simulink model "Questao6_lab3_d"  (R2022b)
settings: Solver=VariableStepAuto  StartTime=0.0  StopTime=43200  RelTol=1e-3
model workspace (MAT data in the model file):
  Cc = 144870
  Ce = 132.0152
  Ci = 959.0196
  Rai = 10.1213
  Rca = 0.0037
  Rcp = 0.0021
  Rec = 0.7046
  Rei = 0.3194
  gamma = 0.021
libraries: simulink x1
settings Model: Creator=pedro  LastModifiedBy=pedro

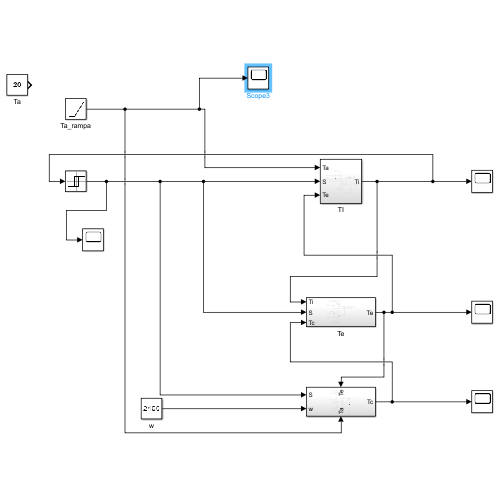
[thumbnail: Simulink's stored preview of the top-level diagram]
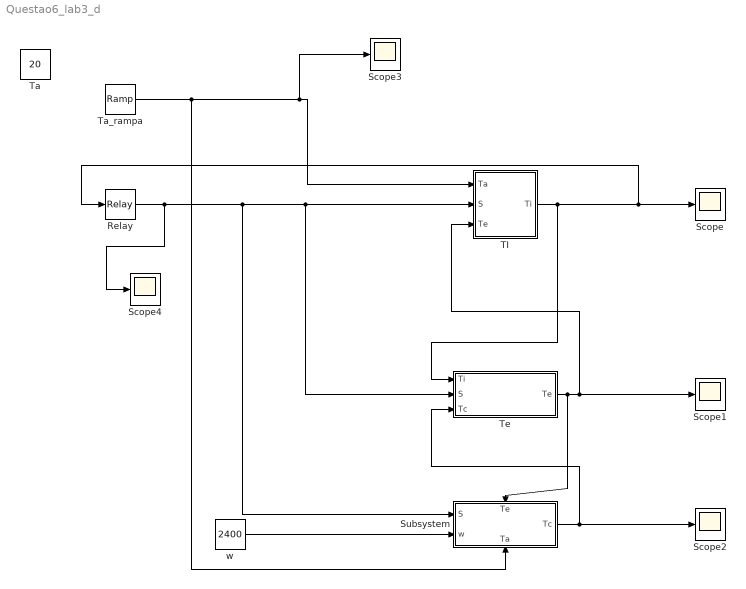
== system Questao6_lab3_d ==
  Relay : Relay  OnSwitchValue=-18  OffSwitchValue=-22
  Scope{,1..4} (5 alike) : Scope
  Subsystem : Subsystem
      settings: PortSchema="{\"entries\":[{\"content\":{\"sides\":[{\"content\":{\"connectorIds\":[\"In1\",\"In2\"]},\"type\":\"ConnectorPlacement.EquallySpacedRectSide\",\"uuid\":\"e4dc530d-a30f-4d16-a3a8-0b29c322cb05\"},{\"content\":{\"connectorIds\":[\"Out1\"],\"side\":\"RIGHT\"},\"type\":\"ConnectorPlacement.EquallySpacedRectSide\",\"uuid\":\"577ed7dc-9ca1-47d3-813d-dbd0e25e4133\"},{\"content\":{\"connectorIds\":[\"In3\"],\"side\":\"TOP\"},\"type\":\"ConnectorPlacement.EquallySpacedRectSide\",\"uuid\":\"620c9041-5bc5-42ec-a8b0-b7d9c339b1cc\"},{\"content\":{\"connectorIds\":[\"In4\"],\"side\":\"BOTTOM\"},\"type\":\"ConnectorPlacement.EquallySpacedRectSide\",\"uuid\":\"ef1172fe-f891-4bcf-86d4-e4c409d11709\"}]},\"type\":\"ConnectorPlacement.EquallySpacedConnector\",\"uuid\":\"e83013fb-e5b3-4752-857f-b18005700dfb\"}],\"packageUris\":[\"http://schema.mathworks.com/mf0/Connector/R2020b\"],\"version\":\"1.0\"}"
  TI : Subsystem
  Ta : Constant  Value=20
  Ta_rampa : simulink/Sources/Ramp  slope=0.0004629623148  start=0  InitialOutput=20
  Te : Subsystem
  w : Constant  Value=2400
  wires:
  Relay/1 -> Scope4/1, Subsystem/1(S), Te/2(S), TI/2(S)
  Te/1(Te) -> TI/3(Te), Scope1/1, Subsystem/3(Te)
  TI/1(Ti) -> Te/1(Ti), Relay/1, Scope/1
  Subsystem/1(Tc) -> Te/3(Tc), Scope2/1
  w/1 -> Subsystem/2(w)
  Ta_rampa/1 -> Scope3/1, TI/1(Ta), Subsystem/4(Ta)

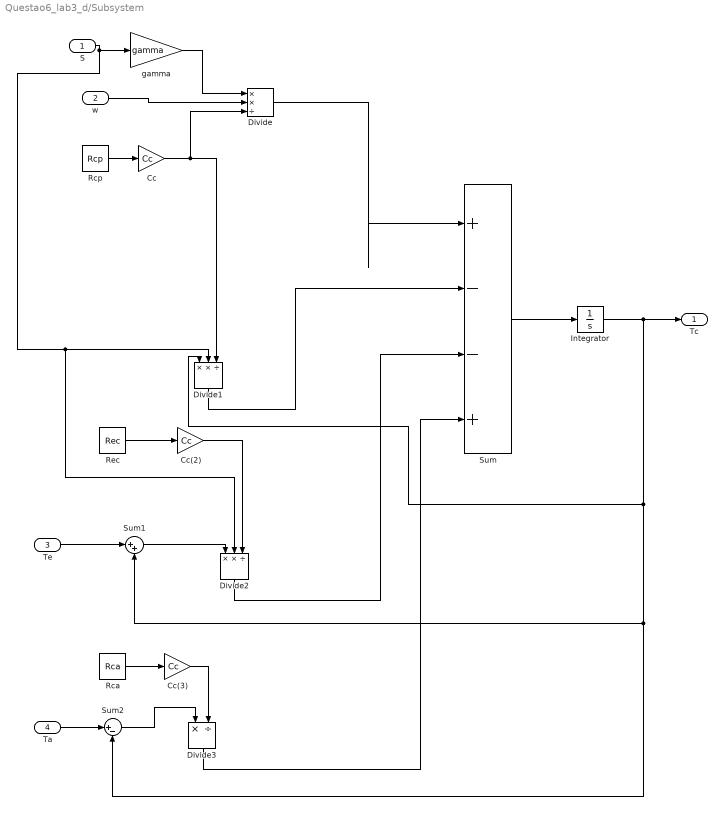
== system Questao6_lab3_d/Subsystem ==
  S : Inport
  w : Inport  Port=2
  Te : Inport  Port=3
  Ta : Inport  Port=4
  Cc : Gain  Gain=Cc
  Cc(2) : Gain  Gain=Cc
  Cc(3) : Gain  Gain=Cc
  Divide : Product  Inputs=**/
  Divide1 : Product  Inputs=**/
  Divide2 : Product  Inputs=**/
  Divide3 : Product  Inputs=*/
  Integrator : Integrator
  Rca : Constant  Value=Rca
  Rcp : Constant  Value=Rcp
  Rec : Constant  Value=Rec
  Sum : Sum  Inputs=|+--+
  Sum1 : Sum  Inputs=|++
  Sum2 : Sum  Inputs=|+-
  gamma : Gain  Gain=gamma
  Tc : Outport
  wires:
  S/1 -> gamma/1, Divide1/2, Divide2/2
  gamma/1 -> Divide/1
  w/1 -> Divide/2
  Rcp/1 -> Cc/1
  Cc/1 -> Divide1/3, Divide/3
  Divide/1 -> Sum/1
  Divide1/1 -> Sum/2
  Te/1 -> Sum1/1
  Sum1/1 -> Divide2/1
  Rec/1 -> Cc(2)/1
  Cc(2)/1 -> Divide2/3
  Divide2/1 -> Sum/3
  Rca/1 -> Cc(3)/1
  Ta/1 -> Sum2/1
  Sum2/1 -> Divide3/1
  Cc(3)/1 -> Divide3/2
  Divide3/1 -> Sum/4
  Sum/1 -> Integrator/1
  Integrator/1 -> Divide1/1, Sum1/2, Sum2/2, Tc/1

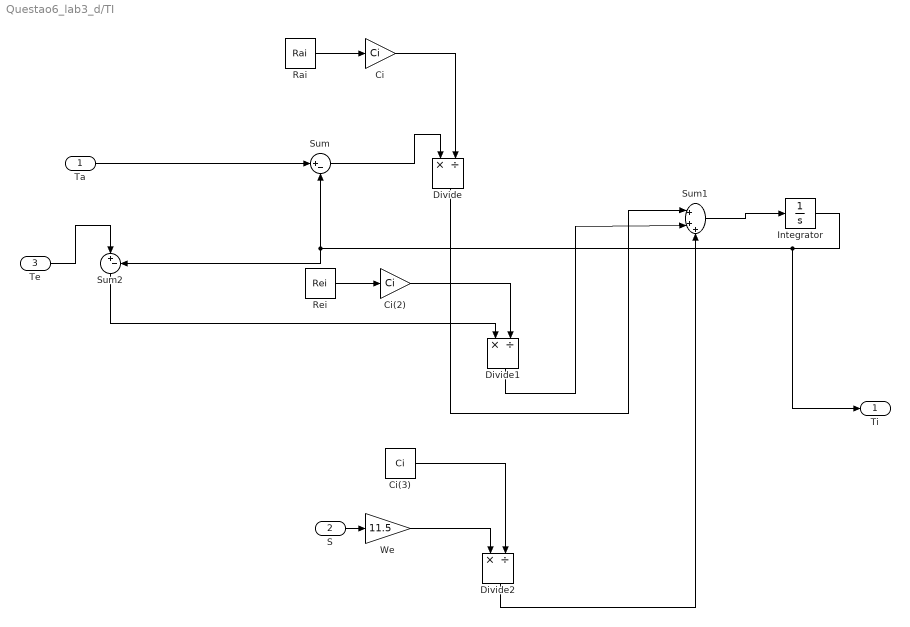
== system Questao6_lab3_d/TI ==
  Ta : Inport
  S : Inport  Port=2
  Te : Inport  Port=3
  Ci : Gain  Gain=Ci
  Ci(2) : Gain  Gain=Ci
  Ci(3) : Constant  Value=Ci
  Divide : Product  Inputs=*/
  Divide1 : Product  Inputs=*/
  Divide2 : Product  Inputs=*/
  Integrator : Integrator  InitialCondition=20
  Rai : Constant  Value=Rai
  Rei : Constant  Value=Rei
  Sum : Sum  Inputs=|+-
  Sum1 : Sum  Inputs=|+++
  Sum2 : Sum  Inputs=|+-
  We : Gain  Gain=11.5
  Ti : Outport
  wires:
  S/1 -> We/1
  Ci/1 -> Divide/2
  Divide/1 -> Sum1/1
  Sum1/1 -> Integrator/1
  Ci(2)/1 -> Divide1/2
  Integrator/1 -> Sum/2, Sum2/2, Ti/1
  Ci(3)/1 -> Divide2/2
  We/1 -> Divide2/1
  Divide2/1 -> Sum1/3
  Rai/1 -> Ci/1
  Sum/1 -> Divide/1
  Divide1/1 -> Sum1/2
  Rei/1 -> Ci(2)/1
  Sum2/1 -> Divide1/1
  Ta/1 -> Sum/1
  Te/1 -> Sum2/1

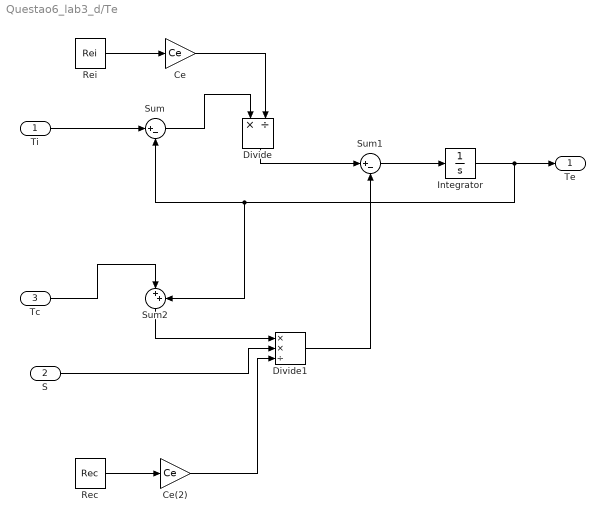
== system Questao6_lab3_d/Te ==
  Ti : Inport
  S : Inport  Port=2
  Tc : Inport  Port=3
  Ce : Gain  Gain=Ce
  Ce(2) : Gain  Gain=Ce
  Divide : Product  Inputs=*/
  Divide1 : Product  Inputs=**/
  Integrator : Integrator
  Rec : Constant  Value=Rec
  Rei : Constant  Value=Rei
  Sum : Sum  Inputs=|+-
  Sum1 : Sum  Inputs=|+-
  Sum2 : Sum  Inputs=|++
  Te : Outport
  wires:
  Ti/1 -> Sum/1
  Sum/1 -> Divide/1
  Rei/1 -> Ce/1
  Ce/1 -> Divide/2
  Divide/1 -> Sum1/1
  Tc/1 -> Sum2/1
  Sum2/1 -> Divide1/1
  S/1 -> Divide1/2
  Rec/1 -> Ce(2)/1
  Ce(2)/1 -> Divide1/3
  Divide1/1 -> Sum1/2
  Sum1/1 -> Integrator/1
  Integrator/1 -> Sum2/2, Sum/2, Te/1
